simulink model "exampl_leg_wheel"  (R2024a)
settings: Solver=FixedStepAuto  StartTime=0.0  StopTime=10.0  FixedStep=0.0001  RelTol=1e-3
values from neighbouring files (symbols this model uses):
  K = lqr(A,B,Q,R)    [example.m]
  N = mp*{x2+L*(-theta1*sin(theta)+theta2*cos(theta))}+Nm    [example.m]
undefined symbols (not defined in the file or in its folder): X, Y, Z
libraries: sm_lib x69, nesl_utility x28, slpidlib x5
(part 1 of 3)
settings Model: Creator=lenovo  LastModifiedBy=lenovo
settings SolverCC: ZeroCrossAlgorithm=Adaptive
settings DebuggingCC: IgnoredZcDiagnostic=none  UnconnectedInputMsg=warning  UnconnectedOutputMsg=warning  UnconnectedLineMsg=warning  UnderSpecifiedDimensionMsg=warning
settings ModelReferenceCC: EnableRefExpFcnMdlSchedulingChecks=on
settings RTWCC: GPUComputeCapability=3.5  DLArmComputeVersion=19.05

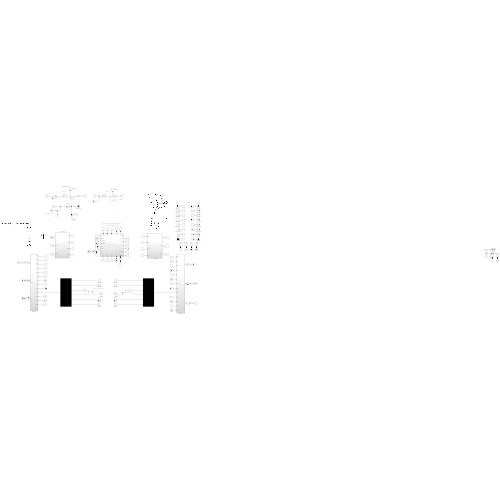
[thumbnail: Simulink's stored preview of the top-level diagram]
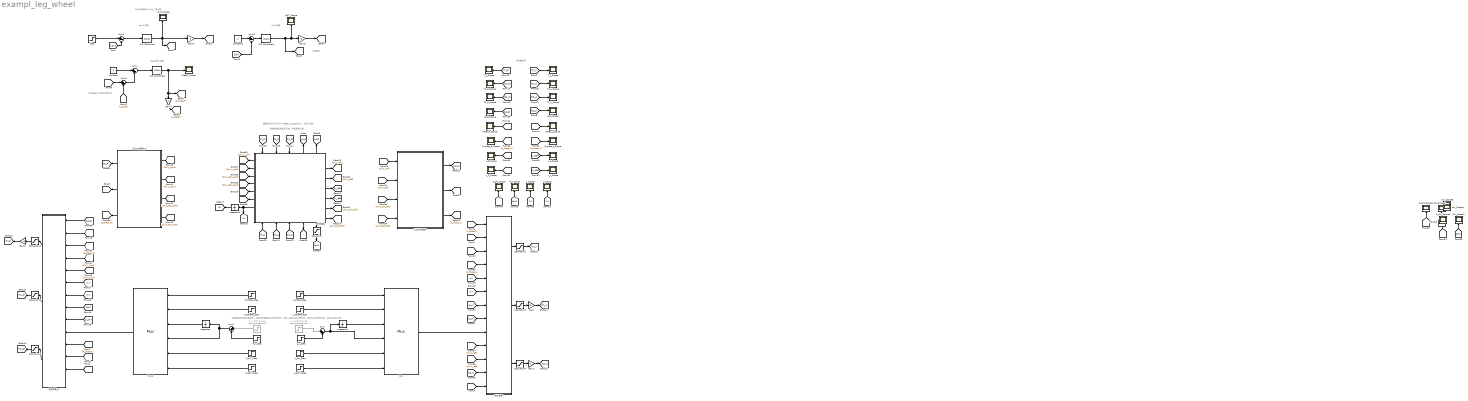
== system exampl_leg_wheel ==
  note: 向左边转输出的yaw_T是正数
  note: 需要先在命令行运行 K=get_k_length(0.2)，算出K矩阵
  note: 这里期望位移是轮速积分，会比机体速度积分出来的值大，因此x起到正向加速作用，实际不会这样写代码，实物以实际为准。
  note: 中间量观测
  note: theta角补偿器
  note: roll补偿器
  note: yaw补偿器
  note: 用角度制观测是否正确，用弧度制计算。
  note: theta_error是右边减左边
  note: 右侧取负
  Constant : Constant  Value=0
  Constant1 : Constant  Value=0
  Gain{,1..4,6} (6 alike) : Gain  Gain=-1
  Integrator : Integrator
  Integrator1 : Integrator
  Integrator3 : Integrator
  L0_L_Scope : Scope
  L0_R_Scope : Scope
  L_dphi_Step : Step  Time=0  After=0  SampleTime=0
  L_dtheta_Step : Step  Time=0  After=0  SampleTime=0
  L_phi_Step : Step  Time=0  After=0  SampleTime=0
  L_theta_Step : Step  Time=0  After=0  SampleTime=0
  L_v_Step : Step  Time=0.5  After=1.2  SampleTime=0
  L_v_Stepchange : Step  Commented=on  Time=6  After=-1  SampleTime=0
  Mux : Mux  Inputs=6
  Mux1 : Mux  Inputs=6
  PID Controller : slpidlib/PID Controller  Controller=PID  Form=Parallel  TimeDomain=Continuous-time  UseExternalTs=off  SampleTime=-1  IntegratorMethod=Forward Euler  FilterMethod=Forward Euler  ControllerParametersSource=internal  P=1  I=0  UseKiTs=off  D=0.5  UseExternalDerivativeSource=off  N=100  UseFilter=on  TunerSelectOption=Transfer Function Based (PID Tuner App)  InitialConditionSource=internal  InitialConditionForIntegrator=0  InitialConditionForFilter=0  DifferentiatorICPrevScaledInput=0  ExternalReset=none  TrackingMode=off  Kt=1  LimitOutput=off  SatLimitsSource=internal  UpperSaturationLimit=inf  LowerSaturationLimit=-inf  LinearizeAsGain=on  AntiWindupMode=none  Kb=1  LimitIntegrator=off  UpperIntegratorSaturationLimit=inf  LowerIntegratorSaturationLimit=-inf  POutMin=[]  POutMax=[]  IOutMin=[]  IOutMax=[]  DOutMin=[]  DOutMax=[]  NOutMin=[]  NOutMax=[]  SumOutMin=[]  SumOutMax=[]  SaturationOutMin=[]  SaturationOutMax=[]  PParamMin=[]  PParamMax=[]  IParamMin=[]  IParamMax=[]  DParamMin=[]  DParamMax=[]  NParamMin=[]  NParamMax=[]  KbParamMin=[]  KbParamMax=[]  KtParamMin=[]  KtParamMax=[]  KbOutMin=[]  KbOutMax=[]  KtOutMin=[]  KtOutMax=[]  IntegratorOutMin=[]  IntegratorOutMax=[]  FilterOutMin=[]  FilterOutMax=[]  SumI1OutMin=[]  SumI1OutMax=[]  SumI2OutMin=[]  SumI2OutMax=[]  SumI3OutMin=[]  SumI3OutMax=[]  SumI4OutMin=[]  SumI4OutMax=[]  SumDOutMin=[]  SumDOutMax=[]  DifferentiatorOutMin=[]  DifferentiatorOutMax=[]  FilterDiffOutCoefMin=[]  FilterDiffOutCoefMax=[]  ReciprocalOutMin=[]  ReciprocalOutMax=[]  SumDenOutMin=[]  SumDenOutMax=[]  SumNumOutMin=[]  SumNumOutMax=[]  DivideOutMin=[]  DivideOutMax=[]  UdiffTsProdOutMin=[]  UdiffTsProdOutMax=[]  NTsProdOutMin=[]  NTsProdOutMax=[]  UintegralTsProdOutMin=[]  UintegralTsProdOutMax=[]  UngainTsProdOutMin=[]  UngainTsProdOutMax=[]  ClampingZeroOutDataTypeStr=Inherit: Inherit via back propagation  ClampingZeroOutMin=[]  ClampingZeroOutMax=[]  FilterDenConstantOutDataTypeStr=Inherit: Inherit via back propagation  FilterDenConstantOutMin=[]  FilterDenConstantOutMax=[]  PCopyOutDataTypeStr=Inherit: Inherit via back propagation  PCopyOutMin=[]  PCopyOutMax=[]  NCopyOutDataTypeStr=Inherit: Inherit via back propagation  NCopyOutMin=[]  NCopyOutMax=[]  IntegratorContinuousStateAttributes=''  IntegratorStateMustResolveToSignalObject=off  IntegratorRTWStateStorageClass=Auto  FilterContinuousStateAttributes=''  FilterStateMustResolveToSignalObject=off  FilterRTWStateStorageClass=Auto  ParallelPVariant=InternalParameters  IdealPVariant=Disabled  IVariant=InternalParameters  DVariant=InternalParameters  IntegratorVariant=Continuous  SatVariant=Disabled  AWVariant=Passthrough  PCopyVariant=Disabled  TRVariant=Disabled  FdbkBlocksVariant=Forward  IdealPFdbkVariant=Disabled  SatFdbkVariant=Disabled  DerivativeFilterVariant=ContFilter  NVariant=InternalParameters  NCopyVariant=Disabled  FilterICVariant=InternalICsFilter  IntegratorICVariant=InternalICs  ExternalResetVariant=Disabled  TRSumVariant=Passthrough  SumFdbkVariant=Disabled  SumVariant=Sum_PID  TsampFilterVariant=InternalTs  TsampNgainVariant=Passthrough  TsampIntegralVariant=Disabled_SignalSpec  ExternalSaturationOutDataTypeStr=Inherit: Same as second input  DerivativeSourceVariant=ErrorSignal
  PID Controller1 : slpidlib/PID Controller  Controller=PID  Form=Parallel  TimeDomain=Continuous-time  UseExternalTs=off  SampleTime=-1  IntegratorMethod=Forward Euler  FilterMethod=Forward Euler  ControllerParametersSource=internal  P=100  I=0  UseKiTs=off  D=30  UseExternalDerivativeSource=off  N=100  UseFilter=on  TunerSelectOption=Transfer Function Based (PID Tuner App)  InitialConditionSource=internal  InitialConditionForIntegrator=0  InitialConditionForFilter=0  DifferentiatorICPrevScaledInput=0  ExternalReset=none  TrackingMode=off  Kt=1  LimitOutput=off  SatLimitsSource=internal  UpperSaturationLimit=inf  LowerSaturationLimit=-inf  LinearizeAsGain=on  AntiWindupMode=none  Kb=1  LimitIntegrator=off  UpperIntegratorSaturationLimit=inf  LowerIntegratorSaturationLimit=-inf  POutMin=[]  POutMax=[]  IOutMin=[]  IOutMax=[]  DOutMin=[]  DOutMax=[]  NOutMin=[]  NOutMax=[]  SumOutMin=[]  SumOutMax=[]  SaturationOutMin=[]  SaturationOutMax=[]  PParamMin=[]  PParamMax=[]  IParamMin=[]  IParamMax=[]  DParamMin=[]  DParamMax=[]  NParamMin=[]  NParamMax=[]  KbParamMin=[]  KbParamMax=[]  KtParamMin=[]  KtParamMax=[]  KbOutMin=[]  KbOutMax=[]  KtOutMin=[]  KtOutMax=[]  IntegratorOutMin=[]  IntegratorOutMax=[]  FilterOutMin=[]  FilterOutMax=[]  SumI1OutMin=[]  SumI1OutMax=[]  SumI2OutMin=[]  SumI2OutMax=[]  SumI3OutMin=[]  SumI3OutMax=[]  SumI4OutMin=[]  SumI4OutMax=[]  SumDOutMin=[]  SumDOutMax=[]  DifferentiatorOutMin=[]  DifferentiatorOutMax=[]  FilterDiffOutCoefMin=[]  FilterDiffOutCoefMax=[]  ReciprocalOutMin=[]  ReciprocalOutMax=[]  SumDenOutMin=[]  SumDenOutMax=[]  SumNumOutMin=[]  SumNumOutMax=[]  DivideOutMin=[]  DivideOutMax=[]  UdiffTsProdOutMin=[]  UdiffTsProdOutMax=[]  NTsProdOutMin=[]  NTsProdOutMax=[]  UintegralTsProdOutMin=[]  UintegralTsProdOutMax=[]  UngainTsProdOutMin=[]  UngainTsProdOutMax=[]  ClampingZeroOutDataTypeStr=Inherit: Inherit via back propagation  ClampingZeroOutMin=[]  ClampingZeroOutMax=[]  FilterDenConstantOutDataTypeStr=Inherit: Inherit via back propagation  FilterDenConstantOutMin=[]  FilterDenConstantOutMax=[]  PCopyOutDataTypeStr=Inherit: Inherit via back propagation  PCopyOutMin=[]  PCopyOutMax=[]  NCopyOutDataTypeStr=Inherit: Inherit via back propagation  NCopyOutMin=[]  NCopyOutMax=[]  IntegratorContinuousStateAttributes=''  IntegratorStateMustResolveToSignalObject=off  IntegratorRTWStateStorageClass=Auto  FilterContinuousStateAttributes=''  FilterStateMustResolveToSignalObject=off  FilterRTWStateStorageClass=Auto  ParallelPVariant=InternalParameters  IdealPVariant=Disabled  IVariant=InternalParameters  DVariant=InternalParameters  IntegratorVariant=Continuous  SatVariant=Disabled  AWVariant=Passthrough  PCopyVariant=Disabled  TRVariant=Disabled  FdbkBlocksVariant=Forward  IdealPFdbkVariant=Disabled  SatFdbkVariant=Disabled  DerivativeFilterVariant=ContFilter  NVariant=InternalParameters  NCopyVariant=Disabled  FilterICVariant=InternalICsFilter  IntegratorICVariant=InternalICs  ExternalResetVariant=Disabled  TRSumVariant=Passthrough  SumFdbkVariant=Disabled  SumVariant=Sum_PID  TsampFilterVariant=InternalTs  TsampNgainVariant=Passthrough  TsampIntegralVariant=Disabled_SignalSpec  ExternalSaturationOutDataTypeStr=Inherit: Same as second input  DerivativeSourceVariant=ErrorSignal
  PID Controller2 : slpidlib/PID Controller  Controller=PID  Form=Parallel  TimeDomain=Continuous-time  UseExternalTs=off  SampleTime=-1  IntegratorMethod=Forward Euler  FilterMethod=Forward Euler  ControllerParametersSource=internal  P=100  I=0  UseKiTs=off  D=30  UseExternalDerivativeSource=off  N=100  UseFilter=on  TunerSelectOption=Transfer Function Based (PID Tuner App)  InitialConditionSource=internal  InitialConditionForIntegrator=0  InitialConditionForFilter=0  DifferentiatorICPrevScaledInput=0  ExternalReset=none  TrackingMode=off  Kt=1  LimitOutput=off  SatLimitsSource=internal  UpperSaturationLimit=inf  LowerSaturationLimit=-inf  LinearizeAsGain=on  AntiWindupMode=none  Kb=1  LimitIntegrator=off  UpperIntegratorSaturationLimit=inf  LowerIntegratorSaturationLimit=-inf  POutMin=[]  POutMax=[]  IOutMin=[]  IOutMax=[]  DOutMin=[]  DOutMax=[]  NOutMin=[]  NOutMax=[]  SumOutMin=[]  SumOutMax=[]  SaturationOutMin=[]  SaturationOutMax=[]  PParamMin=[]  PParamMax=[]  IParamMin=[]  IParamMax=[]  DParamMin=[]  DParamMax=[]  NParamMin=[]  NParamMax=[]  KbParamMin=[]  KbParamMax=[]  KtParamMin=[]  KtParamMax=[]  KbOutMin=[]  KbOutMax=[]  KtOutMin=[]  KtOutMax=[]  IntegratorOutMin=[]  IntegratorOutMax=[]  FilterOutMin=[]  FilterOutMax=[]  SumI1OutMin=[]  SumI1OutMax=[]  SumI2OutMin=[]  SumI2OutMax=[]  SumI3OutMin=[]  SumI3OutMax=[]  SumI4OutMin=[]  SumI4OutMax=[]  SumDOutMin=[]  SumDOutMax=[]  DifferentiatorOutMin=[]  DifferentiatorOutMax=[]  FilterDiffOutCoefMin=[]  FilterDiffOutCoefMax=[]  ReciprocalOutMin=[]  ReciprocalOutMax=[]  SumDenOutMin=[]  SumDenOutMax=[]  SumNumOutMin=[]  SumNumOutMax=[]  DivideOutMin=[]  DivideOutMax=[]  UdiffTsProdOutMin=[]  UdiffTsProdOutMax=[]  NTsProdOutMin=[]  NTsProdOutMax=[]  UintegralTsProdOutMin=[]  UintegralTsProdOutMax=[]  UngainTsProdOutMin=[]  UngainTsProdOutMax=[]  ClampingZeroOutDataTypeStr=Inherit: Inherit via back propagation  ClampingZeroOutMin=[]  ClampingZeroOutMax=[]  FilterDenConstantOutDataTypeStr=Inherit: Inherit via back propagation  FilterDenConstantOutMin=[]  FilterDenConstantOutMax=[]  PCopyOutDataTypeStr=Inherit: Inherit via back propagation  PCopyOutMin=[]  PCopyOutMax=[]  NCopyOutDataTypeStr=Inherit: Inherit via back propagation  NCopyOutMin=[]  NCopyOutMax=[]  IntegratorContinuousStateAttributes=''  IntegratorStateMustResolveToSignalObject=off  IntegratorRTWStateStorageClass=Auto  FilterContinuousStateAttributes=''  FilterStateMustResolveToSignalObject=off  FilterRTWStateStorageClass=Auto  ParallelPVariant=InternalParameters  IdealPVariant=Disabled  IVariant=InternalParameters  DVariant=InternalParameters  IntegratorVariant=Continuous  SatVariant=Disabled  AWVariant=Passthrough  PCopyVariant=Disabled  TRVariant=Disabled  FdbkBlocksVariant=Forward  IdealPFdbkVariant=Disabled  SatFdbkVariant=Disabled  DerivativeFilterVariant=ContFilter  NVariant=InternalParameters  NCopyVariant=Disabled  FilterICVariant=InternalICsFilter  IntegratorICVariant=InternalICs  ExternalResetVariant=Disabled  TRSumVariant=Passthrough  SumFdbkVariant=Disabled  SumVariant=Sum_PID  TsampFilterVariant=InternalTs  TsampNgainVariant=Passthrough  TsampIntegralVariant=Disabled_SignalSpec  ExternalSaturationOutDataTypeStr=Inherit: Same as second input  DerivativeSourceVariant=ErrorSignal
  R_dphi_Step : Step  Time=0  After=0  SampleTime=0
  R_dtheta_Step : Step  Time=0  After=0  SampleTime=0
  R_phi_Step : Step  Time=0  After=0  SampleTime=0
  R_theta_Step : Step  Time=0  After=0  SampleTime=0
  R_v_Step : Step  Time=0.5  After=1.2  SampleTime=0
  R_v_Stepchange : Step  Commented=on  Time=6  After=-1  SampleTime=0
  Saturation : Saturate  UpperLimit=pi/2  LowerLimit=-pi/2
  Saturation1 : Saturate  UpperLimit=10  LowerLimit=-10  ZeroCross=off
  Saturation2 : Saturate  UpperLimit=10  LowerLimit=-10
  Saturation{3..6} (4 alike) : Saturate  UpperLimit=100  LowerLimit=-100  ZeroCross=off
  Step : Step  Time=0.3  After=0  SampleTime=0
  Sum : Sum  Inputs=|++
  Sum1 : Sum  Inputs=|++
  Sum{2..5} (4 alike) : Sum  Inputs=|+-
  T1_L_Scope : Scope
  T1_R_Scope : Scope
  T2_L_Scope : Scope
  T2_R_Scope : Scope
  T_L_Scope : Scope
  T_R_Scope : Scope
  d_phi_Scope : Scope
  d_phi_Scope1 : Scope
  d_phi_Scope2 : Scope
  d_theta_L_Scope : Scope
  d_theta_R_Scope : Scope
  phi_Scope{,1..4} (5 alike) : Scope
  rollT_Scope : Scope
  thetaT_Scope : Scope
  theta_L_Scope : Scope
  theta_R_Scope : Scope
  v_L_Scope : Scope
  v_R_Scope : Scope
  v_Scope : Scope
  x_L_Scope : Scope
  x_R_Scope : Scope
  x_Scope : Scope
  yawT_Scope : Scope
  机体模型 : Subsystem
      settings: PortSchema="{\"entries\":[{\"content\":{\"sides\":[{\"content\":{\"connectorIds\":[\"Out12\",\"Out13\",\"Out14\",\"Out15\",\"Out16\",\"Out17\",\"Out18\",\"Out19\"]},\"type\":\"ConnectorPlacement.EquallySpacedRectSide\",\"uuid\":\"4be4cf3c-8d4a-439d-b5cb-06ad5eef59d8\"},{\"content\":{\"connectorIds\":[\"Out1\",\"Out2\",\"Out3\",\"Out4\",\"Out5\",\"Out6\",\"Out7\"],\"side\":\"RIGHT\"},\"type\":\"ConnectorPlacement.EquallySpacedRectSide\",\"uuid\":\"9f385abe-4754-448e-b1c2-da916b327b4e\"},{\"content\":{\"connectorIds\":[\"In1\",\"In2\",\"In3\",\"Out10\",\"Out11\"],\"side\":\"TOP\"},\"type\":\"ConnectorPlacement.EquallySpacedRectSide\",\"uuid\":\"0d7aeff5-6f71-4f4a-9817-d2f8e8297452\"},{\"content\":{\"connectorIds\":[\"In4\",\"In5\",\"In6\",\"Out8\",\"Out9\"],\"side\":\"BOTTOM\"},\"type\":\"ConnectorPlacement.EquallySpacedRectSide\",\"uuid\":\"a7c4e407-434f-4782-96e7-6c585313a74e\"}]},\"type\":\"ConnectorPlacement.EquallySpacedConnector\",\"uuid\":\"6b173a6a-efbd-4e34-a31b-a53ece42b69c\"}],\"packageUris\":[\"http://schema.mathworks.com/mf0/Connector/R2020b\"],\"version\":\"1.0\"}"
  正运动学解算 : Subsystem
  正运动学解算_R : Subsystem
  输出解算 : Subsystem
  输出解算_R : Subsystem
  wires:
  Mux/1 -> 输出解算/9(xd)
  机体模型/9(phi) -> Saturation/1
  正运动学解算/2(theta) -> [L_theta]
  Mux1/1 -> 输出解算_R/10(xd)
  输出解算_R/1(T) -> Saturation2/1
  Saturation2/1 -> Gain2/1
  L_theta_Step/1 -> Mux/1
  L_dtheta_Step/1 -> Mux/2
  L_phi_Step/1 -> Mux/5
  L_dphi_Step/1 -> Mux/6
  R_dtheta_Step/1 -> Mux1/2
  R_dphi_Step/1 -> Mux1/6
  R_theta_Step/1 -> Mux1/1
  R_phi_Step/1 -> Mux1/5
  Sum2/1 -> PID Controller/1
  PID Controller1/1 -> thetaT_Scope/1, [R_thetaT], Gain4/1
  Step/1 -> Sum2/1
  PID Controller/1 -> [R_yawT], yawT_Scope/1, Gain3/1
  正运动学解算_R/2(theta) -> [R_theta]
  Gain3/1 -> [L_yawT]
  [R_yawT] -> 输出解算_R/13(yawT)
  [L_yawT] -> 输出解算/13(yawT)
  [yaw] -> Sum2/2
  机体模型/10(yaw) -> [yaw]
  Saturation3/1 -> Gain/1
  Saturation4/1 -> Gain1/1
  PID Controller2/1 -> [L_rollT], Gain6/1, rollT_Scope/1
  机体模型/11(roll) -> [roll]
  [L_rollT] -> 输出解算/2(rollT)
  [R_rollT] -> 输出解算_R/12(rollT)
  Gain4/1 -> [L_thetaT]
  [R_thetaT] -> 输出解算_R/11(thetaT)
  [L_thetaT] -> 输出解算/1(thetaT)
  [R_theta] -> Sum3/1
  [L_theta] -> Sum3/2
  [L_theta] -> theta_L_Scope/1
  [L_theta] -> 输出解算/3(theta)
  [R_theta] -> 输出解算_R/2(theta)
  [R_theta] -> theta_R_Scope/1
  Saturation6/1 -> [T2_R]
  输出解算_R/3(T2) -> Saturation6/1
  Saturation5/1 -> [T1_R]
  输出解算_R/2(T1) -> Saturation5/1
  [T2_R] -> T2_R_Scope/1
  [T1_R] -> T1_R_Scope/1
  Gain2/1 -> [T_R]
  [T_R] -> T_R_Scope/1
  输出解算/2(T1) -> Saturation3/1
  输出解算/3(T2) -> Saturation4/1
  Gain1/1 -> [T2_L]
  Gain/1 -> [T1_L]
  输出解算/1(T) -> Saturation1/1
  Saturation1/1 -> [T_L]
  [T_L] -> T_L_Scope/1
  [T1_L] -> T1_L_Scope/1
  [T2_L] -> T2_L_Scope/1
  [T_L] -> 机体模型/4(T_L)
  [T1_L] -> 机体模型/5(T1_L)
  [T2_L] -> 机体模型/6(T2_L)
  [T2_R] -> 机体模型/3(T2_R)
  [T1_R] -> 机体模型/2(T1_R)
  [T_R] -> 机体模型/1(T_R)
  机体模型/18(v) -> Integrator3/1, [v]
  Integrator3/1 -> [x]
  [x] -> 输出解算_R/6(x)
  [v] -> 输出解算_R/7(v)
  [x] -> 输出解算/5(x)
  [v] -> 输出解算/6(v)
  Integrator/1 -> Mux1/3
  Integrator1/1 -> Mux/3
  机体模型/16(x_right) -> [x_right]
  机体模型/4(x_left) -> [x_left]
  机体模型/17(v_right) -> [v_right]
  机体模型/5(v_left) -> [v_left]
  [v_left] -> v_L_Scope/1
  [v_right] -> v_R_Scope/1
  机体模型/2(phi1_left) -> [phi1_left]
  机体模型/3(phi4_left) -> [phi4_left]
  [phi4_left] -> 正运动学解算/2(phi4)
  [phi1_left] -> 正运动学解算/1(phi1)
  [phi4_left] -> 输出解算/11(phi4)
  [phi1_left] -> 输出解算/10(phi1)
  机体模型/6(phi1_dot_left) -> [phi1_dot_left]
  机体模型/7(phi4_dot_left) -> [phi4_dot_left]
  [phi1_dot_left] -> 正运动学解算/3(d_phi1)
  [phi4_dot_left] -> 正运动学解算/4(d_phi4)
  机体模型/12(phi1_right) -> [phi1_right]
  机体模型/13(phi4_right) -> [phi4_right]
  机体模型/14(phi1_dot_right) -> [phi1_dot_right]
  机体模型/15(phi4_dot_right) -> [phi4_dot_right]
  [phi1_right] -> 正运动学解算_R/1(phi1)
  [phi4_right] -> 正运动学解算_R/2(phi4)
  [phi1_dot_right] -> 正运动学解算_R/3(d_phi1)
  [phi4_dot_right] -> 正运动学解算_R/4(d_phi4)
  [phi1_right] -> 输出解算_R/4(phi1)
  [phi4_right] -> 输出解算_R/5(phi4)
  机体模型/8(d_phi) -> [d_phi]
  [d_phi] -> 输出解算_R/9(d_phi)
  [d_phi] -> 输出解算/8(d_phi)
  [d_phi] -> d_phi_Scope/1
  Saturation/1 -> [phi]
  [phi] -> 输出解算_R/8(phi)
  [phi] -> 输出解算/7(phi)
  正运动学解算/3(d_theta) -> [d_theta_L]
  正运动学解算/1(L0) -> [L0_L]
  [d_theta_L] -> d_theta_L_Scope/1
  [L0_L] -> 输出解算/12(L0)
  [d_theta_L] -> 输出解算/4(d_theta)
  正运动学解算_R/1(L0) -> [L0_R]
  正运动学解算_R/3(d_theta) -> [d_theta_R]
  [d_theta_R] -> 输出解算_R/3(d_theta)
  [L0_R] -> 输出解算_R/1(L0)
  [d_theta_R] -> d_theta_R_Scope/1
  [L0_L] -> L0_L_Scope/1
  [L0_R] -> L0_R_Scope/1
  [x_right] -> x_R_Scope/1
  [x_left] -> x_L_Scope/1
  [phi] -> phi_Scope/1
  [phi] -> phi_Scope2/1
  [d_phi] -> d_phi_Scope1/1
  [phi] -> phi_Scope1/1
  [d_phi] -> d_phi_Scope2/1
  [x] -> x_Scope/1
  [v] -> v_Scope/1
  L_v_Step/1 -> Sum/2
  Sum/1 -> Integrator1/1, Mux/4
  R_v_Step/1 -> Sum1/2
  L_v_Stepchange/1 -> Sum/1
  R_v_Stepchange/1 -> Sum1/1
  Sum1/1 -> Mux1/4, Integrator/1
  Constant/1 -> Sum4/1
  Sum3/1 -> Sum4/2
  Sum4/1 -> PID Controller1/1
  [roll] -> Sum5/2
  Constant1/1 -> Sum5/1
  Sum5/1 -> PID Controller2/1
  Gain6/1 -> [R_rollT]
